simulink library "Drive_Mode_Librery (1)"  (R2025b)
settings: Solver=VariableStepAuto  StartTime=0.0  StopTime=10.0  RelTol=1e-3

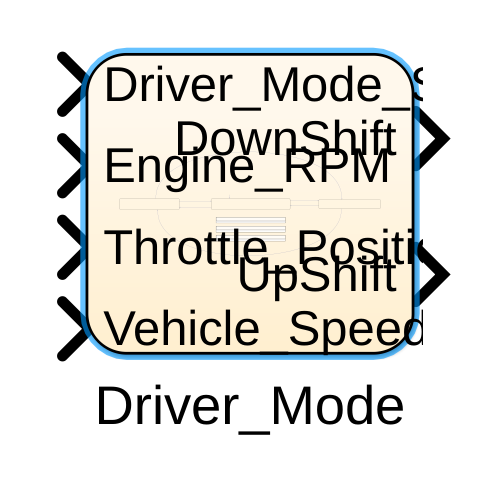
[thumbnail: Simulink's stored preview of the top-level diagram]
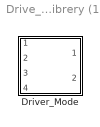
== system Drive_Mode_Librery (1) ==
  Driver_Mode : Stateflow chart  TreatAsAtomicUnit=on

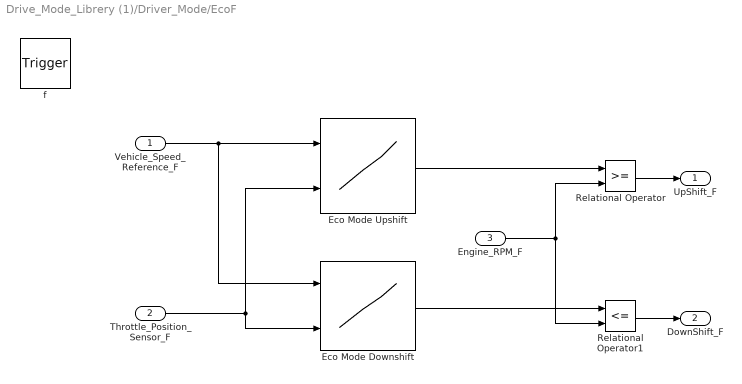
== system Drive_Mode_Librery (1)/Driver_Mode/EcoF ==
  Vehicle_Speed_Reference_F : Inport
  Throttle_Position_Sensor_F : Inport  Port=2
  Engine_RPM_F : Inport  Port=3
  f : TriggerPort  TriggerType=function-call  VariantControl=(inherit)
      settings: CopyFcn=Stateflow.SLINSF.SimulinkMan.removeBlockPreDeleteFcn  PreDeleteFcn=Stateflow.SLINSF.SimulinkMan.unsafePredeleteFcn
  Eco Mode Downshift : Lookup_n-D  BreakpointsForDimension1=[0 20 40 60 80 100 120 140 160 180 200 220 240]  BreakpointsForDimension2=[0 10 20 30 40 50 60 70 80 90 100]  Table=|  InternalRulePriority=Speed  RndMeth=Simplest
      | [900 920 950 1000 1050 1100 1150 1200 1250 1300 1350;
      |  920 940 970 1020 1070 1120 1170 1220 1270 1320 1370;
      |  950 980 1050 1120 1200 1280 1360 1440 1520 1600 1650;
      |  1000 1040 1100 1180 1280 1380 1480 1580 1680 1780 1880;
      |  1100 1140 1220 1320 1440 1560 1680 1800 1920 2040 2160;
      |  1200 1240 1340 1460 1580 1700 1820 1940 2060 2180 2300;
      |  1300 1340 1460 1600 1740 1880 2020 2160 2300 2440 2580;
      |  1400 1440 1580 1740 1900 2060 2220 2380 2540 2700 2860;
      |  1500 1540 1700 1880 2060 2240 2420 2600 2780 2960 3140;
      |  1600 1650 1830 2020 2220 2420 2620 2820 3020 3220 3420;
      |  1800 1860 2060 2270 2490 2710 2930 3150 3370 3590 3810;
      |  2000 2060 2280 2510 2740 2970 3200 3430 3660 3890 4120;
      |  2200 2280 2520 2760 3000 3240 3480 3720 3960 4200 4440]
      settings: InputPortMap=u0,u1
  Eco Mode Upshift : Lookup_n-D  BreakpointsForDimension1=[0 20 40 60 80 100 120 140 160 180 200 220 240]  BreakpointsForDimension2=[0 10 20 30 40 50 60 70 80 90 100]  Table=|  InternalRulePriority=Speed  RndMeth=Simplest
      | [1200 1250 1300 1350 1400 1450 1500 1550 1600 1650 1700;
      |  1250 1300 1350 1400 1450 1500 1550 1600 1650 1700 1750;
      |  1300 1350 1420 1500 1580 1660 1740 1820 1900 1980 2050;
      |  1400 1450 1550 1650 1760 1870 1980 2090 2200 2310 2400;
      |  1500 1550 1670 1790 1930 2070 2220 2370 2520 2670 2820;
      |  1600 1680 1820 1970 2130 2300 2470 2640 2810 2980 3150;
      |  1700 1800 1960 2130 2310 2490 2680 2870 3060 3250 3440;
      |  1850 1960 2140 2330 2530 2740 2960 3180 3400 3620 3840;
      |  2000 2130 2330 2540 2760 2980 3210 3440 3670 3900 4130;
      |  2200 2340 2560 2790 3030 3270 3520 3770 4020 4270 4520;
      |  2400 2560 2800 3050 3310 3570 3840 4110 4380 4650 4920;
      |  2600 2780 3040 3310 3590 3870 4160 4450 4740 5030 5320;
      |  2800 3000 3280 3560 3850 4140 4440 4740 5040 5340 5640]
      settings: InputPortMap=u0,u1
  Relational Operator : RelationalOperator  OutDataTypeStr=boolean  RndMeth=Simplest  InputSameDT=off
  Relational Operator1 : RelationalOperator  Operator=<=  OutDataTypeStr=boolean  RndMeth=Simplest  InputSameDT=off
  UpShift_F : Outport
  DownShift_F : Outport  Port=2
  wires:
  Eco Mode Upshift/1 -> Relational Operator/1
  Throttle_Position_Sensor_F/1 -> Eco Mode Downshift/2, Eco Mode Upshift/2
  Relational Operator/1 -> UpShift_F/1
  Engine_RPM_F/1 -> Relational Operator1/2, Relational Operator/2
  Relational Operator1/1 -> DownShift_F/1
  Eco Mode Downshift/1 -> Relational Operator1/1
  Vehicle_Speed_Reference_F/1 -> Eco Mode Downshift/1, Eco Mode Upshift/1

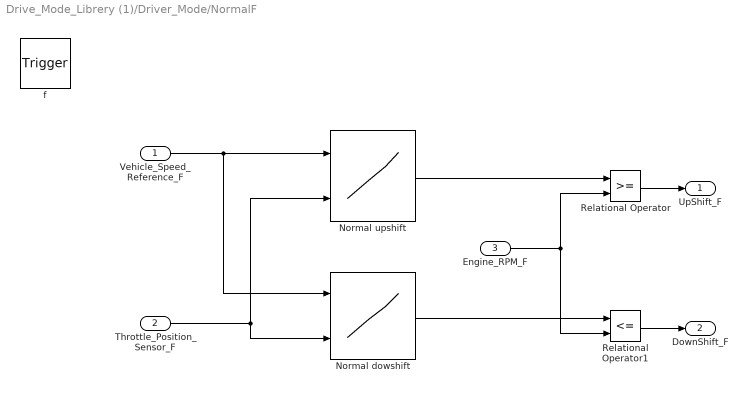
== system Drive_Mode_Librery (1)/Driver_Mode/NormalF ==
  Vehicle_Speed_Reference_F : Inport
  Throttle_Position_Sensor_F : Inport  Port=2
  Engine_RPM_F : Inport  Port=3
  f : TriggerPort  TriggerType=function-call  VariantControl=(inherit)
      settings: CopyFcn=Stateflow.SLINSF.SimulinkMan.removeBlockPreDeleteFcn  PreDeleteFcn=Stateflow.SLINSF.SimulinkMan.unsafePredeleteFcn
  Normal dowshift : Lookup_n-D  BreakpointsForDimension1=[0 20 40 60 80 100 120 140 160 180 200 220 240]  BreakpointsForDimension2=[0 10 20 30 40 50 60 70 80 90 100]  Table=|  InternalRulePriority=Speed  RndMeth=Simplest
      | [1000 1040 1100 1180 1260 1340 1420 1500 1580 1660 1740;
      |  1040 1080 1140 1220 1300 1380 1460 1540 1620 1700 1780;
      |  1100 1160 1240 1320 1400 1480 1560 1640 1720 1800 1880;
      |  1180 1240 1340 1440 1540 1640 1740 1840 1940 2040 2140;
      |  1260 1340 1440 1560 1680 1800 1920 2040 2160 2280 2400;
      |  1360 1440 1560 1680 1800 1920 2040 2160 2280 2400 2520;
      |  1480 1560 1680 1820 1960 2100 2240 2380 2520 2660 2800;
      |  1600 1680 1820 1960 2100 2240 2380 2520 2660 2800 2940;
      |  1740 1840 1980 2120 2260 2400 2540 2680 2820 2960 3100;
      |  1880 2000 2160 2320 2480 2640 2800 2960 3120 3280 3440;
      |  2040 2180 2360 2540 2720 2900 3080 3260 3440 3620 3800;
      |  2200 2360 2540 2720 2900 3080 3260 3440 3620 3800 3980;
      |  2380 2560 2760 2960 3160 3360 3560 3760 3960 4160 4360]
      settings: InputPortMap=u0,u1
  Normal upshift : Lookup_n-D  BreakpointsForDimension1=[0 20 40 60 80 100 120 140 160 180 200 220 240]  BreakpointsForDimension2=[0 10 20 30 40 50 60 70 80 90 100]  Table=|  InternalRulePriority=Speed  RndMeth=Simplest
      | [1500 1600 1700 1800 1900 2000 2100 2200 2300 2400 2500;
      |  1600 1700 1800 1920 2040 2160 2280 2400 2520 2640 2760;
      |  1700 1820 1960 2100 2240 2380 2520 2660 2800 2940 3080;
      |  1820 1940 2100 2260 2420 2580 2740 2900 3060 3220 3380;
      |  1950 2080 2260 2440 2620 2800 2980 3160 3340 3520 3700;
      |  2100 2240 2440 2640 2840 3040 3240 3440 3640 3840 4040;
      |  2260 2420 2640 2860 3080 3300 3520 3740 3960 4180 4400;
      |  2440 2620 2860 3100 3340 3580 3820 4060 4300 4540 4780;
      |  2620 2820 3080 3340 3600 3860 4120 4380 4640 4900 5160;
      |  2820 3040 3320 3600 3880 4160 4440 4720 5000 5280 5560;
      |  3040 3280 3580 3880 4180 4480 4780 5080 5380 5680 5980;
      |  3260 3520 3840 4160 4480 4800 5120 5440 5760 6080 6400;
      |  3500 3780 4120 4460 4800 5140 5480 5820 6160 6500 6840]
      settings: InputPortMap=u0,u1
  Relational Operator : RelationalOperator  OutDataTypeStr=boolean  RndMeth=Simplest  InputSameDT=off
  Relational Operator1 : RelationalOperator  Operator=<=  OutDataTypeStr=boolean  RndMeth=Simplest  InputSameDT=off
  UpShift_F : Outport
  DownShift_F : Outport  Port=2
  wires:
  Normal dowshift/1 -> Relational Operator1/1
  Throttle_Position_Sensor_F/1 -> Normal dowshift/2, Normal upshift/2
  Normal upshift/1 -> Relational Operator/1
  Relational Operator/1 -> UpShift_F/1
  Engine_RPM_F/1 -> Relational Operator1/2, Relational Operator/2
  Vehicle_Speed_Reference_F/1 -> Normal dowshift/1, Normal upshift/1
  Relational Operator1/1 -> DownShift_F/1

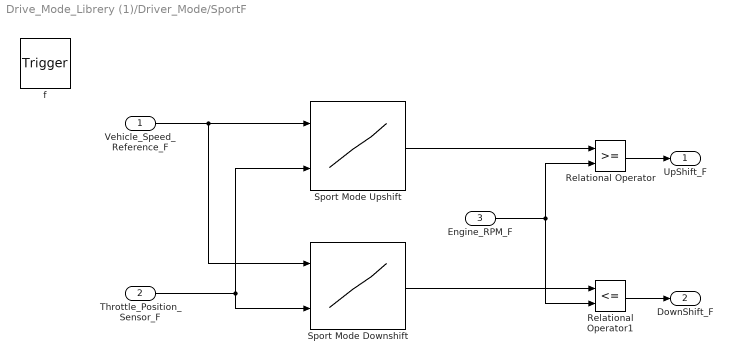
== system Drive_Mode_Librery (1)/Driver_Mode/SportF ==
  Vehicle_Speed_Reference_F : Inport
  Throttle_Position_Sensor_F : Inport  Port=2
  Engine_RPM_F : Inport  Port=3
  f : TriggerPort  TriggerType=function-call  VariantControl=(inherit)
      settings: CopyFcn=Stateflow.SLINSF.SimulinkMan.removeBlockPreDeleteFcn  PreDeleteFcn=Stateflow.SLINSF.SimulinkMan.unsafePredeleteFcn
  Relational Operator : RelationalOperator  OutDataTypeStr=boolean  RndMeth=Simplest  InputSameDT=off
  Relational Operator1 : RelationalOperator  Operator=<=  OutDataTypeStr=boolean  RndMeth=Simplest  InputSameDT=off
  Sport Mode Downshift : Lookup_n-D  BreakpointsForDimension1=[0 20 40 60 80 100 120 140 160 180 200 220 240]  BreakpointsForDimension2=[0 10 20 30 40 50 60 70 80 90 100]  Table=|  InternalRulePriority=Speed  RndMeth=Simplest
      | [900 950 1000 1150 1300 1450 1600 1750 1900 2050 2200;
      |  950 1000 1150 1300 1450 1600 1750 1900 2050 2200 2350;
      |  1000 1150 1300 1450 1600 1750 1900 2050 2200 2350 2500;
      |  1150 1300 1450 1600 1750 1900 2050 2200 2350 2500 2650;
      |  1300 1450 1600 1750 1900 2050 2200 2350 2500 2650 2800;
      |  1450 1600 1750 1900 2050 2200 2400 2600 2800 3000 3200;
      |  1600 1750 1900 2050 2200 2400 2600 2800 3000 3200 3400;
      |  1750 1900 2050 2200 2350 2600 2850 3050 3250 3450 3650;
      |  1900 2050 2200 2350 2500 2750 3050 3300 3550 3800 4000;
      |  2050 2200 2350 2500 2700 2950 3250 3550 3850 4100 4350;
      |  2200 2350 2500 2650 2850 3100 3400 3700 4000 4250 4500;
      |  2350 2500 2650 2800 3000 3300 3600 3950 4250 4550 4850;
      |  2500 2650 2800 2950 3150 3450 3750 4100 4400 4700 5000]
      settings: InputPortMap=u0,u1
  Sport Mode Upshift : Lookup_n-D  BreakpointsForDimension1=[0 20 40 60 80 100 120 140 160 180 200 220 240]  BreakpointsForDimension2=[0 10 20 30 40 50 60 70 80 90 100]  Table=|  InternalRulePriority=Speed  RndMeth=Simplest
      | [1700 1850 2000 2150 2300 2450 2600 2750 2900 3050 3200;
      |  1850 2000 2150 2300 2450 2600 2750 2900 3050 3200 3350;
      |  2000 2150 2300 2450 2600 2750 2900 3050 3200 3350 3500;
      |  2150 2300 2450 2600 2750 2900 3050 3200 3350 3500 3650;
      |  2300 2450 2600 2750 2900 3050 3200 3350 3500 3650 3800;
      |  2450 2600 2750 2900 3050 3200 3400 3600 3800 4000 4200;
      |  2600 2750 2900 3050 3200 3400 3600 3800 4000 4200 4400;
      |  2750 2900 3050 3200 3350 3600 3850 4050 4250 4450 4650;
      |  2900 3050 3200 3350 3500 3750 4050 4300 4550 4800 5000;
      |  3050 3200 3350 3500 3700 3950 4250 4550 4850 5100 5350;
      |  3200 3350 3500 3650 3850 4100 4400 4700 5000 5300 5600;
      |  3350 3500 3650 3800 4000 4300 4600 4950 5250 5550 5850;
      |  3500 3650 3800 3950 4200 4500 4850 5200 5550 5850 6150]
      settings: InputPortMap=u0,u1
  UpShift_F : Outport
  DownShift_F : Outport  Port=2
  wires:
  Sport Mode Downshift/1 -> Relational Operator1/1
  Throttle_Position_Sensor_F/1 -> Sport Mode Downshift/2, Sport Mode Upshift/2
  Sport Mode Upshift/1 -> Relational Operator/1
  Relational Operator/1 -> UpShift_F/1
  Engine_RPM_F/1 -> Relational Operator1/2, Relational Operator/2
  Vehicle_Speed_Reference_F/1 -> Sport Mode Downshift/1, Sport Mode Upshift/1
  Relational Operator1/1 -> DownShift_F/1

== stateflow chart Drive_Mode_Librery (1)/Driver_Mode ==
  state Eco
    during:
    [UpShift,DownShift] = EcoF(Vehicle_Speed_Reference,Throttle_Position_Sensor,Engine_RPM)
  state Normal
    during:
    [UpShift,DownShift] = NormalF(Vehicle_Speed_Reference,Throttle_Position_Sensor,Engine_RPM)
  state Sport
    during:
    [UpShift,DownShift] = SportF(Vehicle_Speed_Reference,Throttle_Position_Sensor,Engine_RPM)
  state [UpShift_F,DownShift_F] = EcoF(Vehicle_Speed_Reference_F,Throttle_Position_Sensor_F,Engine_RPM_F) [function]
  state [UpShift_F,DownShift_F] = NormalF(Vehicle_Speed_Reference_F,Throttle_Position_Sensor_F,Engine_RPM_F) [function]
  state [UpShift_F,DownShift_F] = SportF(Vehicle_Speed_Reference_F,Throttle_Position_Sensor_F,Engine_RPM_F) [function]
  Eco -> Sport [order 2] : [Driver_Mode_Selection == 1]
  (default) -> Normal
  Normal -> Sport [order 2] : [Driver_Mode_Selection == 1]
  Eco -> Normal [order 1] : [Driver_Mode_Selection == 2]
  Sport -> Normal [order 1] : [Driver_Mode_Selection == 2]
  Normal -> Eco [order 1] : [Driver_Mode_Selection == 0]
  Sport -> Eco [order 2] : [Driver_Mode_Selection == 0]
  data: Vehicle_Speed_Reference_F function_input; Throttle_Position_Sensor_F function_input; UpShift_F function_output; DownShift_F function_output; Engine_RPM_F function_input; Vehicle_Speed_Reference_F function_input; Throttle_Position_Sensor_F function_input; Engine_RPM_F function_input; UpShift_F function_output; DownShift_F function_output; Vehicle_Speed_Reference_F function_input; Throttle_Position_Sensor_F function_input; Engine_RPM_F function_input; UpShift_F function_output; DownShift_F function_output; Driver_Mode_Selection input uint8 size=1; Engine_RPM input uint16 size=1; Throttle_Position_Sensor input uint8 size=1; Vehicle_Speed_Reference input uint8 size=1; DownShift output uint8 size=1; UpShift output uint8 size=1
